simulink model "TST_CoVeh_SpdCoord"  (R2016b)
settings: Solver=FixedStepDiscrete  StartTime=0.0  StopTime=simTime  FixedStep=sampleTime  RelTol=1e-3
values from neighbouring files (symbols this model uses):
  testCase = 1    [initTST_CoVeh_SpdCoord_001.m]
libraries: simulink x2
settings Model: Creator=WF305  LastModifiedBy=WF305
settings DebuggingCC: SignalRangeChecking=error

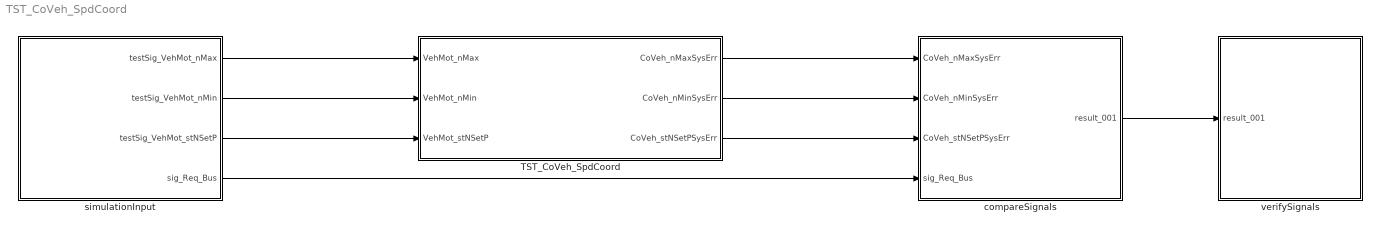
== system TST_CoVeh_SpdCoord ==
  TST_CoVeh_SpdCoord : Subsystem
  compareSignals : Subsystem
  simulationInput : Subsystem
  verifySignals : Subsystem
  wires:
  simulationInput/1(testSig_VehMot_nMax) -> TST_CoVeh_SpdCoord/1(VehMot_nMax)
  simulationInput/2(testSig_VehMot_nMin) -> TST_CoVeh_SpdCoord/2(VehMot_nMin)
  simulationInput/3(testSig_VehMot_stNSetP) -> TST_CoVeh_SpdCoord/3(VehMot_stNSetP)
  TST_CoVeh_SpdCoord/1(CoVeh_nMaxSysErr) -> compareSignals/1(CoVeh_nMaxSysErr)
  TST_CoVeh_SpdCoord/2(CoVeh_nMinSysErr) -> compareSignals/2(CoVeh_nMinSysErr)
  TST_CoVeh_SpdCoord/3(CoVeh_stNSetPSysErr) -> compareSignals/3(CoVeh_stNSetPSysErr)
  simulationInput/4(sig_Req_Bus) -> compareSignals/4(sig_Req_Bus)
  compareSignals/1(result_001) -> verifySignals/1(result_001)

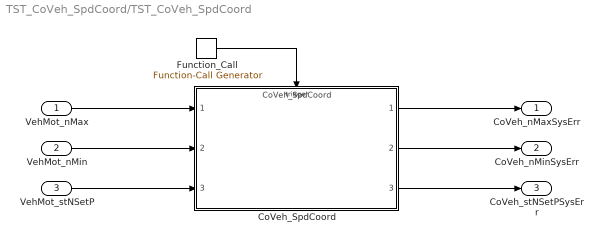
== system TST_CoVeh_SpdCoord/TST_CoVeh_SpdCoord ==
  VehMot_nMax : Inport
  VehMot_nMin : Inport  Port=2
  VehMot_stNSetP : Inport  Port=3
  CoVeh_SpdCoord : ModelReference  ModelNameDialog=CoVeh_SpdCoord  ModelReferenceVersion=1.5  TriggerPortName=function  TriggerPortTriggerType=function-call  TriggerPortStatesWhenEnabling=held
  Function_Call : simulink/Ports & Subsystems/Function-Call Generator  sample_time=sampleTime  numberOfIterations=1
  CoVeh_nMaxSysErr : Outport
  CoVeh_nMinSysErr : Outport  Port=2
  CoVeh_stNSetPSysErr : Outport  Port=3
  wires:
  Function_Call/1 -> CoVeh_SpdCoord/Trigger
  VehMot_nMax/1 -> CoVeh_SpdCoord/1
  VehMot_nMin/1 -> CoVeh_SpdCoord/2
  VehMot_stNSetP/1 -> CoVeh_SpdCoord/3
  CoVeh_SpdCoord/1 -> CoVeh_nMaxSysErr/1
  CoVeh_SpdCoord/2 -> CoVeh_nMinSysErr/1
  CoVeh_SpdCoord/3 -> CoVeh_stNSetPSysErr/1

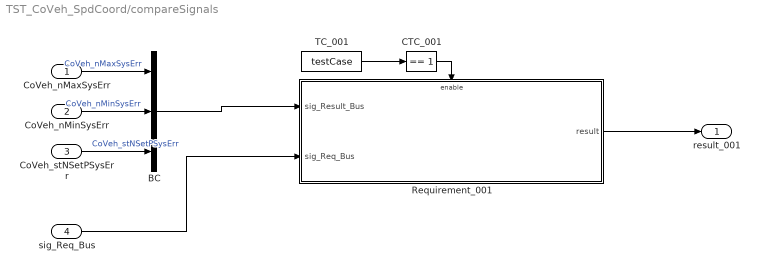
== system TST_CoVeh_SpdCoord/compareSignals ==
  CoVeh_nMaxSysErr : Inport
  CoVeh_nMinSysErr : Inport  Port=2
  CoVeh_stNSetPSysErr : Inport  Port=3
  sig_Req_Bus : Inport  Port=4
  BC : BusCreator  Inputs=3
  CTC_001 : simulink/Logic and Bit Operations/Compare To Constant  relop===  const=1  OutDataTypeStr=boolean
  Requirement_001 : Subsystem
  TC_001 : Constant  Value=testCase
  result_001 : Outport
  wires:
  CoVeh_nMaxSysErr/1 -> BC/1  "CoVeh_nMaxSysErr"
  CoVeh_nMinSysErr/1 -> BC/2  "CoVeh_nMinSysErr"
  CoVeh_stNSetPSysErr/1 -> BC/3  "CoVeh_stNSetPSysErr"
  TC_001/1 -> CTC_001/1
  CTC_001/1 -> Requirement_001/Enable
  sig_Req_Bus/1 -> Requirement_001/2(sig_Req_Bus)
  BC/1 -> Requirement_001/1(sig_Result_Bus)
  Requirement_001/1(result) -> result_001/1

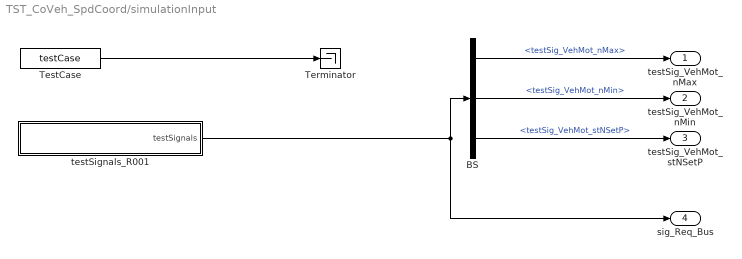
== system TST_CoVeh_SpdCoord/simulationInput ==
  BS : BusSelector  OutputSignals=testSig_VehMot_nMax,testSig_VehMot_nMin,testSig_VehMot_stNSetP
  Terminator : Terminator
  TestCase : Constant  Value=testCase
  testSignals_R001 : Subsystem
  testSig_VehMot_nMax : Outport
  testSig_VehMot_nMin : Outport  Port=2
  testSig_VehMot_stNSetP : Outport  Port=3
  sig_Req_Bus : Outport  Port=4
  wires:
  BS/1 -> testSig_VehMot_nMax/1  "<testSig_VehMot_nMax>"
  BS/2 -> testSig_VehMot_nMin/1  "<testSig_VehMot_nMin>"
  BS/3 -> testSig_VehMot_stNSetP/1  "<testSig_VehMot_stNSetP>"
  testSignals_R001/1(testSignals) -> BS/1, sig_Req_Bus/1
  TestCase/1 -> Terminator/1

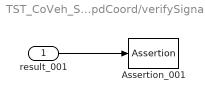
== system TST_CoVeh_SpdCoord/verifySignals ==
  result_001 : Inport
  Assertion_001 : Assertion
  wires:
  result_001/1 -> Assertion_001/1

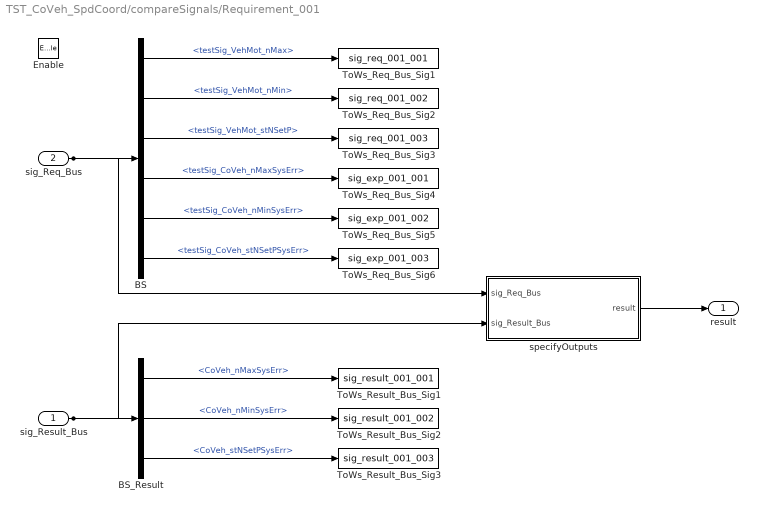
== system TST_CoVeh_SpdCoord/compareSignals/Requirement_001 ==
  sig_Result_Bus : Inport
  sig_Req_Bus : Inport  Port=2
  Enable : EnablePort
  BS : BusSelector  OutputSignals=testSig_VehMot_nMax,testSig_VehMot_nMin,testSig_VehMot_stNSetP,testSig_CoVeh_nMaxSysErr,testSig_CoVeh_nMinSysErr,testSig_CoVeh_stNSetPSysErr
  BS_Result : BusSelector  OutputSignals=CoVeh_nMaxSysErr,CoVeh_nMinSysErr,CoVeh_stNSetPSysErr
  ToWs_Req_Bus_Sig1 : ToWorkspace  VariableName=sig_req_001_001  SaveFormat=Structure With Time
  ToWs_Req_Bus_Sig2 : ToWorkspace  VariableName=sig_req_001_002  SaveFormat=Structure With Time
  ToWs_Req_Bus_Sig3 : ToWorkspace  VariableName=sig_req_001_003  SaveFormat=Structure With Time
  ToWs_Req_Bus_Sig4 : ToWorkspace  VariableName=sig_exp_001_001  SaveFormat=Structure With Time
  ToWs_Req_Bus_Sig5 : ToWorkspace  VariableName=sig_exp_001_002  SaveFormat=Structure With Time
  ToWs_Req_Bus_Sig6 : ToWorkspace  VariableName=sig_exp_001_003  SaveFormat=Structure With Time
  ToWs_Result_Bus_Sig1 : ToWorkspace  VariableName=sig_result_001_001  SaveFormat=Structure With Time
  ToWs_Result_Bus_Sig2 : ToWorkspace  VariableName=sig_result_001_002  SaveFormat=Structure With Time
  ToWs_Result_Bus_Sig3 : ToWorkspace  VariableName=sig_result_001_003  SaveFormat=Structure With Time
  specifyOutputs : Subsystem
  result : Outport
  wires:
  sig_Req_Bus/1 -> BS/1, specifyOutputs/1(sig_Req_Bus)
  BS/1 -> ToWs_Req_Bus_Sig1/1  "<testSig_VehMot_nMax>"
  BS/2 -> ToWs_Req_Bus_Sig2/1  "<testSig_VehMot_nMin>"
  BS/3 -> ToWs_Req_Bus_Sig3/1  "<testSig_VehMot_stNSetP>"
  BS/4 -> ToWs_Req_Bus_Sig4/1  "<testSig_CoVeh_nMaxSysErr>"
  BS/5 -> ToWs_Req_Bus_Sig5/1  "<testSig_CoVeh_nMinSysErr>"
  BS/6 -> ToWs_Req_Bus_Sig6/1  "<testSig_CoVeh_stNSetPSysErr>"
  sig_Result_Bus/1 -> BS_Result/1, specifyOutputs/2(sig_Result_Bus)
  BS_Result/1 -> ToWs_Result_Bus_Sig1/1  "<CoVeh_nMaxSysErr>"
  BS_Result/2 -> ToWs_Result_Bus_Sig2/1  "<CoVeh_nMinSysErr>"
  BS_Result/3 -> ToWs_Result_Bus_Sig3/1  "<CoVeh_stNSetPSysErr>"
  specifyOutputs/1(result) -> result/1

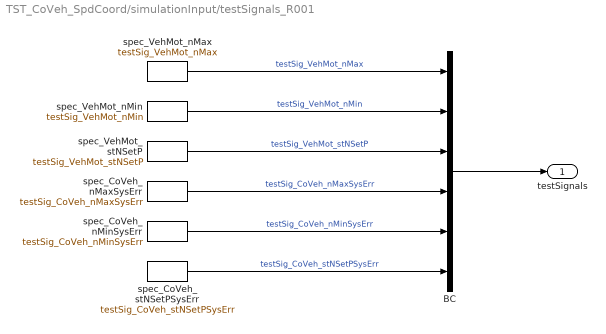
== system TST_CoVeh_SpdCoord/simulationInput/testSignals_R001 ==
  BC : BusCreator  Inputs=6
  spec_CoVeh_nMaxSysErr : FromWorkspace  VariableName=testSig_CoVeh_nMaxSysErr  Interpolate=off  OutputAfterFinalValue=Holding final value
  spec_CoVeh_nMinSysErr : FromWorkspace  VariableName=testSig_CoVeh_nMinSysErr  Interpolate=off  OutputAfterFinalValue=Holding final value
  spec_CoVeh_stNSetPSysErr : FromWorkspace  VariableName=testSig_CoVeh_stNSetPSysErr  Interpolate=off  OutputAfterFinalValue=Holding final value
  spec_VehMot_nMax : FromWorkspace  VariableName=testSig_VehMot_nMax  Interpolate=off  OutputAfterFinalValue=Holding final value
  spec_VehMot_nMin : FromWorkspace  VariableName=testSig_VehMot_nMin  Interpolate=off  OutputAfterFinalValue=Holding final value
  spec_VehMot_stNSetP : FromWorkspace  VariableName=testSig_VehMot_stNSetP  Interpolate=off  OutputAfterFinalValue=Holding final value
  testSignals : Outport
  wires:
  BC/1 -> testSignals/1
  spec_VehMot_nMax/1 -> BC/1  "testSig_VehMot_nMax"
  spec_VehMot_nMin/1 -> BC/2  "testSig_VehMot_nMin"
  spec_VehMot_stNSetP/1 -> BC/3  "testSig_VehMot_stNSetP"
  spec_CoVeh_nMaxSysErr/1 -> BC/4  "testSig_CoVeh_nMaxSysErr"
  spec_CoVeh_nMinSysErr/1 -> BC/5  "testSig_CoVeh_nMinSysErr"
  spec_CoVeh_stNSetPSysErr/1 -> BC/6  "testSig_CoVeh_stNSetPSysErr"

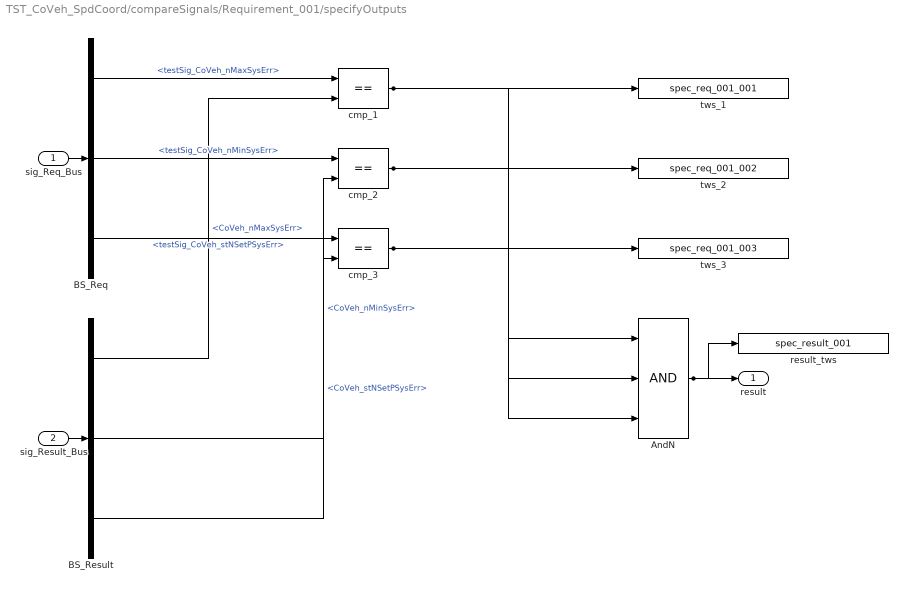
== system TST_CoVeh_SpdCoord/compareSignals/Requirement_001/specifyOutputs ==
  sig_Req_Bus : Inport
  sig_Result_Bus : Inport  Port=2
  AndN : Logic  Inputs=3
  BS_Req : BusSelector  OutputSignals=testSig_CoVeh_nMaxSysErr,testSig_CoVeh_nMinSysErr,testSig_CoVeh_stNSetPSysErr
  BS_Result : BusSelector  OutputSignals=CoVeh_nMaxSysErr,CoVeh_nMinSysErr,CoVeh_stNSetPSysErr
  cmp_1 : RelationalOperator  Operator===  RndMeth=Nearest  InputSameDT=on
  cmp_2 : RelationalOperator  Operator===  RndMeth=Nearest  InputSameDT=on
  cmp_3 : RelationalOperator  Operator===  RndMeth=Nearest  InputSameDT=on
  result_tws : ToWorkspace  VariableName=spec_result_001
  tws_1 : ToWorkspace  VariableName=spec_req_001_001
  tws_2 : ToWorkspace  VariableName=spec_req_001_002
  tws_3 : ToWorkspace  VariableName=spec_req_001_003
  result : Outport
  wires:
  sig_Req_Bus/1 -> BS_Req/1
  sig_Result_Bus/1 -> BS_Result/1
  AndN/1 -> result/1, result_tws/1
  BS_Req/1 -> cmp_1/1  "<testSig_CoVeh_nMaxSysErr>"
  BS_Result/1 -> cmp_1/2  "<CoVeh_nMaxSysErr>"
  cmp_1/1 -> tws_1/1, AndN/1
  BS_Req/2 -> cmp_2/1  "<testSig_CoVeh_nMinSysErr>"
  BS_Result/2 -> cmp_2/2  "<CoVeh_nMinSysErr>"
  cmp_2/1 -> tws_2/1, AndN/2
  BS_Req/3 -> cmp_3/1  "<testSig_CoVeh_stNSetPSysErr>"
  BS_Result/3 -> cmp_3/2  "<CoVeh_stNSetPSysErr>"
  cmp_3/1 -> tws_3/1, AndN/3
